simulink model "Active_seat_04_OFFLINE"  (R2017a)
settings: Solver=ode4  StartTime=0.0  StopTime=25  FixedStep=0.005  RelTol=1e-3  EnableMultiTasking=on
undefined symbols (not defined in the file or in its folder): sigbuilder_block
libraries: simulink x8
settings Model: Creator=Stefano  LastModifiedBy=giulio
settings DataIOCC: LimitDataPoints=on
settings OptimizationCC: LifeSpan=inf
settings DebuggingCC: AllowSymbolicDim=off  SFUnexpectedBacktrackingDiag=warning  SFNoUnconditionalDefaultTransitionDiag=warning  SFExecutionAtInitializationDiag=none
settings ModelReferenceCC: PropagateSignalLabelsOutOfModel=off
settings GRTTargetCC: TargetLangStandard=C89/C90 (ANSI)
settings ConfigComp: CovMetricSettings=dw  CovHtmlReporting=on  CovSaveCumulativeToWorkspaceVar=on  CovSaveSingleToWorkspaceVar=on  CovExternalEMLEnable=off

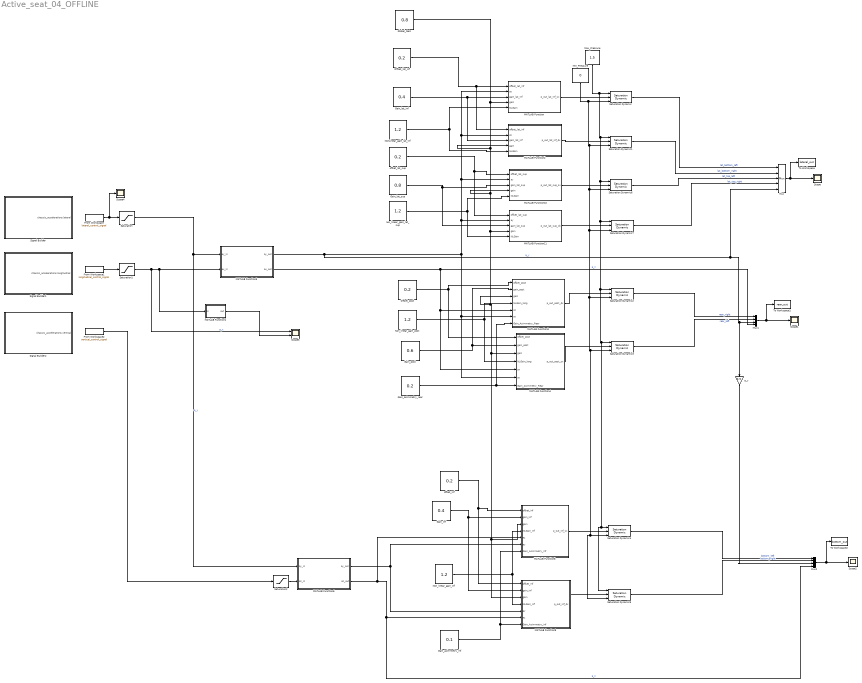
== system Active_seat_04_OFFLINE ==
  From Workspace : FromWorkspace  VariableName=lateral_control_signal  SampleTime=0
  From Workspace1 : FromWorkspace  VariableName=longitudinal_control_signal  SampleTime=0
  From Workspace2 : FromWorkspace  VariableName=vertical_control_signal  SampleTime=0
  Gain_asimmetry_inf : Constant  Value=0.1
  Gain_asimmetry_rear : Constant  Value=0.2
  Gain_inf : Constant  Value=0.4
  Gain_lat_inf : Constant  Value=0.4
  Gain_lat_sup : Constant  Value=0.8
  Gain_post : Constant  Value=0.6
  Global_Gain : Constant  Value=0.8
  MATLAB Function : MATLAB Function  TreatAsAtomicUnit=on
  MATLAB Function1 : MATLAB Function  TreatAsAtomicUnit=on
  MATLAB Function10 : MATLAB Function  TreatAsAtomicUnit=on
  MATLAB Function11 : MATLAB Function  TreatAsAtomicUnit=on
  MATLAB Function2 : MATLAB Function  TreatAsAtomicUnit=on
  MATLAB Function3 : MATLAB Function  TreatAsAtomicUnit=on
  MATLAB Function4 : MATLAB Function  TreatAsAtomicUnit=on
  MATLAB Function5 : MATLAB Function  TreatAsAtomicUnit=on
  MATLAB Function6 : MATLAB Function  TreatAsAtomicUnit=on
  MATLAB Function8 : MATLAB Function  TreatAsAtomicUnit=on
  MATLAB Function9 : MATLAB Function  TreatAsAtomicUnit=on
  Max_Pressure : Constant  Value=1.5
  Min_Pressure : Constant  Value=0
  Mux : Mux  Inputs=5
  Mux1 : Mux
  Mux2 : Mux
  NonLinear_gain_lat_inf : Constant  Value=1.2
  Non_linear_gain_inf : Constant  Value=1.2
  Non_linear_gain_post : Constant  Value=1.2
  Offset_lat_inf : Constant  Value=0.2
  Offset_post : Constant  Value=0.2
  Saturation : Saturate  UpperLimit=5  LowerLimit=-5
  Saturation Dynamic{,1..7} (8 alike) : simulink/Discontinuities/Saturation Dynamic  OutMin=[]  OutMax=[]  OutDataTypeStr=Inherit: Same as second input  OutDataType=fixdt(1, 16)  OutScaling=2^-10  DoSatur=off
  Saturation1 : Saturate  UpperLimit=5  LowerLimit=-5
  Saturation2 : Saturate  UpperLimit=5  LowerLimit=-5
  Scope{,1..2,4} (4 alike) : Scope
  Scope3 : Scope  NumInputPorts=2
  Signal Builder : Subsystem  Tag=STV Subsys  LoadFcn=sigbuilder_block('load');  StartFcn=sigbuilder_block('start');  StopFcn=sigbuilder_block('stop');  ClipboardFcn=sigbuilder_block('clipboard');  mask(Sigbuilder block){tuvar=[0:10]}
      mask help: Simulink:masks:SigbuilderBlock_MD
      mask init:
      | if ~strcmp(get_param(bdroot(gcbh),'SimulationStatus'),'stopped') tuvar = sigbuilder_block('maskInit'); end
      settings: CopyFcn=sigbuilder_block('copy');  DeleteFcn=sigbuilder_block('delete');  ModelCloseFcn=sigbuilder_block('modelClose');  PreSaveFcn=sigbuilder_block('preSave');  PauseFcn=sigbuilder_block('pause');  ContinueFcn=sigbuilder_block('continue');  NameChangeFcn=sigbuilder_block('namechange');  OpenFcn=sigbuilder_block('open',[333 123 550.8 400.2 ]);  CloseFcn=sigbuilder_block('close');
      mask Display: plot(0, 0, 100, 100,[2, 2, 32, 32, 2], [68, 8, 8, 68, 68],[32, 2], [38, 38], [32, 19, 2],[53, 60, 44], [32, 17, 17, 2],[16, 16, 31, 31]);txt = getActiveGroup(gcbh);text(2, 100, txt,'verticalAlignment', 'top');
  Signal Builder1 : Subsystem  Tag=STV Subsys  LoadFcn=sigbuilder_block('load');  StartFcn=sigbuilder_block('start');  StopFcn=sigbuilder_block('stop');  ClipboardFcn=sigbuilder_block('clipboard');  mask(Sigbuilder block){tuvar=[0:10]}
      mask help: Simulink:masks:SigbuilderBlock_MD
      mask init:
      | if ~strcmp(get_param(bdroot(gcbh),'SimulationStatus'),'stopped') tuvar = sigbuilder_block('maskInit'); end
      settings: CopyFcn=sigbuilder_block('copy');  DeleteFcn=sigbuilder_block('delete');  ModelCloseFcn=sigbuilder_block('modelClose');  PreSaveFcn=sigbuilder_block('preSave');  PauseFcn=sigbuilder_block('pause');  ContinueFcn=sigbuilder_block('continue');  NameChangeFcn=sigbuilder_block('namechange');  OpenFcn=sigbuilder_block('open',[333 123 550.8 400.2 ]);  CloseFcn=sigbuilder_block('close');
      mask Display: plot(0, 0, 100, 100,[2, 2, 32, 32, 2], [68, 8, 8, 68, 68],[32, 2], [38, 38], [32, 19, 2],[53, 60, 44], [32, 17, 17, 2],[16, 16, 31, 31]);txt = getActiveGroup(gcbh);text(2, 100, txt,'verticalAlignment', 'top');
  Signal Builder2 : Subsystem  Tag=STV Subsys  LoadFcn=sigbuilder_block('load');  StartFcn=sigbuilder_block('start');  StopFcn=sigbuilder_block('stop');  ClipboardFcn=sigbuilder_block('clipboard');  mask(Sigbuilder block){tuvar=[0:10]}
      mask help: Simulink:masks:SigbuilderBlock_MD
      mask init:
      | if ~strcmp(get_param(bdroot(gcbh),'SimulationStatus'),'stopped') tuvar = sigbuilder_block('maskInit'); end
      settings: CopyFcn=sigbuilder_block('copy');  DeleteFcn=sigbuilder_block('delete');  ModelCloseFcn=sigbuilder_block('modelClose');  PreSaveFcn=sigbuilder_block('preSave');  PauseFcn=sigbuilder_block('pause');  ContinueFcn=sigbuilder_block('continue');  NameChangeFcn=sigbuilder_block('namechange');  OpenFcn=sigbuilder_block('open',[333 123 550.8 400.2 ]);  CloseFcn=sigbuilder_block('close');
      mask Display: plot(0, 0, 100, 100,[2, 2, 32, 32, 2], [68, 8, 8, 68, 68],[32, 2], [38, 38], [32, 19, 2],[53, 60, 44], [32, 17, 17, 2],[16, 16, 31, 31]);txt = getActiveGroup(gcbh);text(2, 100, txt,'verticalAlignment', 'top');
  To Workspace : ToWorkspace  VariableName=lateral_out  SaveFormat=Structure With Time  SampleTime=-1
  To Workspace1 : ToWorkspace  VariableName=rear_out  SaveFormat=Structure With Time  SampleTime=-1
  To Workspace2 : ToWorkspace  VariableName=bottom_out  SaveFormat=Structure With Time  SampleTime=-1
  a_y : Gain  Gain=0.5
  non_linear_gain_lat_sup : Constant  Value=1.2
  offset_inf : Constant  Value=0.2
  offset_lat_sup : Constant  Value=0.2
  wires:
  MATLAB Function2/1(p_out_lat_inf_dx) -> Saturation Dynamic1/2
  MATLAB Function/1(p_out_lat_inf_sx) -> Saturation Dynamic/2
  MATLAB Function3/1(p_out_post_dx) -> Saturation Dynamic2/2
  MATLAB Function4/1(p_out_post_sx) -> Saturation Dynamic3/2
  Gain_lat_inf/1 -> MATLAB Function2/3(gain_lat_inf), MATLAB Function/3(gain_lat_inf)
  MATLAB Function5/2(ax_out) -> Mux1/4, MATLAB Function4/5(ax), MATLAB Function3/5(ax)  "a_x"
  Gain_post/1 -> MATLAB Function4/2(gain_post), MATLAB Function3/2(gain_post)
  Offset_lat_inf/1 -> MATLAB Function2/1(offset_lat_inf), MATLAB Function/1(offset_lat_inf)
  Offset_post/1 -> MATLAB Function4/1(offset_post), MATLAB Function3/1(offset_post)
  Max_Pressure/1 -> Saturation Dynamic/1, Saturation Dynamic6/1, Saturation Dynamic5/1, Saturation Dynamic4/1, Saturation Dynamic3/1, Saturation Dynamic2/1, Saturation Dynamic7/1, Saturation Dynamic1/1
  Min_Pressure/1 -> Saturation Dynamic5/3, Saturation Dynamic4/3, Saturation Dynamic3/3, Saturation Dynamic2/3, Saturation Dynamic7/3, Saturation Dynamic6/3, Saturation Dynamic1/3, Saturation Dynamic/3
  Global_Gain/1 -> MATLAB Function/4(gain), MATLAB Function2/4(gain), MATLAB Function10/4(gain), MATLAB Function11/4(gain), MATLAB Function4/3(gain), MATLAB Function9/3(gain), MATLAB Function8/3(gain), MATLAB Function3/3(gain)
  NonLinear_gain_lat_inf/1 -> MATLAB Function2/5(NLGain), MATLAB Function/5(NLGain)
  Non_linear_gain_post/1 -> MATLAB Function4/4(NLGain_long), MATLAB Function3/4(NLGain_long)
  MATLAB Function6/1(ay_out) -> MATLAB Function9/5(ay), MATLAB Function8/6(ay)
  MATLAB Function6/2(az_out) -> MATLAB Function9/6(az), Mux2/4, MATLAB Function8/5(az)  "a_z"
  offset_inf/1 -> MATLAB Function9/1(offset_inf), MATLAB Function8/1(offset_inf)
  Gain_inf/1 -> MATLAB Function9/2(gain_inf), MATLAB Function8/2(gain_inf)
  Non_linear_gain_inf/1 -> MATLAB Function9/4(NLGain_inf), MATLAB Function8/4(NLGain_inf)
  MATLAB Function8/1(p_out_inf_sx) -> Saturation Dynamic4/2
  MATLAB Function9/1(p_out_inf_dx) -> Saturation Dynamic5/2
  Saturation Dynamic/1 -> Mux/1  "lat_bottom_left"
  Gain_asimmetry_rear/1 -> MATLAB Function4/7(Gain_Asimmetry_Rear), MATLAB Function3/7(Gain_Asimmetry_Rear)
  Gain_asimmetry_inf/1 -> MATLAB Function9/7(Gain_Asimmetry_Inf), MATLAB Function8/7(Gain_Asimmetry_Inf)
  offset_lat_sup/1 -> MATLAB Function11/1(offset_lat_sup), MATLAB Function10/1(offset_lat_sup)
  Gain_lat_sup/1 -> MATLAB Function11/3(gain_lat_sup), MATLAB Function10/3(gain_lat_sup)
  non_linear_gain_lat_sup/1 -> MATLAB Function11/5(NLGain), MATLAB Function10/5(NLGain)
  MATLAB Function10/1(p_out_lat_sup_sx) -> Saturation Dynamic6/2
  MATLAB Function11/1(p_out_lat_sup_dx) -> Saturation Dynamic7/2
  Saturation Dynamic6/1 -> Mux/3  "lat_top_left"
  Saturation Dynamic3/1 -> Mux1/2  "rear_left"
  Saturation Dynamic2/1 -> Mux1/1  "rear_right"
  Saturation Dynamic7/1 -> Mux/4  "lat_top_right"
  Saturation Dynamic1/1 -> Mux/2  "lat_bottom_right"
  Saturation2/1 -> MATLAB Function6/2(az_in)
  MATLAB Function5/1(ay_out) -> Mux/5, a_y/1, Mux1/3, MATLAB Function11/2(ay), MATLAB Function10/2(ay), MATLAB Function2/2(ay), MATLAB Function/2(ay), MATLAB Function4/6(ay), MATLAB Function3/6(ay)  "a_y"
  Saturation Dynamic5/1 -> Mux2/2  "bottom_right"
  Saturation Dynamic4/1 -> Mux2/1  "bottom_left"
  Mux/1 -> To Workspace/1, Scope/1
  Mux1/1 -> To Workspace1/1, Scope1/1
  Mux2/1 -> To Workspace2/1, Scope2/1
  Saturation1/1 -> Scope3/1, MATLAB Function1/1(in), MATLAB Function5/2(ax_in)  "a_x"
  Saturation/1 -> MATLAB Function5/1(ay_in), MATLAB Function6/1(ay_in)  "a_y"
  a_y/1 -> Mux2/3
  MATLAB Function1/1(out) -> Scope3/2
  From Workspace/1 -> Scope4/1, Saturation/1
  From Workspace1/1 -> Saturation1/1
  From Workspace2/1 -> Saturation2/1

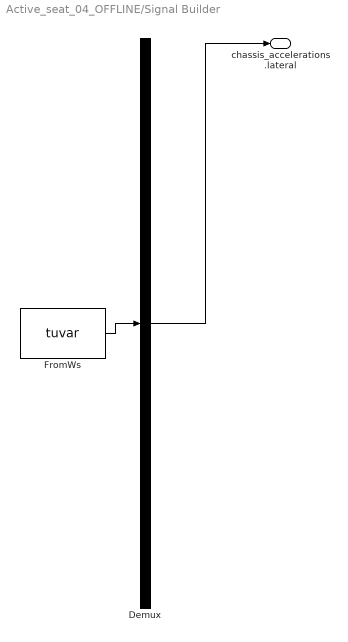
== system Active_seat_04_OFFLINE/Signal Builder ==
  Demux : Demux  Tag=STV Demux  Outputs=1
  FromWs : FromWorkspace  Tag=STV FromWs  VariableName=tuvar  SampleTime=0
      SigBuilderData=|
      | common.afterFinalStr = 'Extrapolate'
      | common.sampleTime = 0
      | dataSet.timeRange = [0 20]
      | dataSet.name = 'Sheet2'
      | sbobj.Name = 'Signal Builder'
      | sbobj.Groups.Name = 'Sheet2'
      | sbobj.Groups.Signals.Name = 'chassis_accelerations.lateral'
      | sbobj.Groups.Signals.XData = [0 0.01 0.02 0.03 0.04 0.05 0.06 0.07 0.08 0.09 0.1 0.11 ... (2001 elements, 1x2001)]
      | sbobj.Groups.Signals.YData = [0.000478634655 0.000129276232 3.6072942e-05 -2.112549e-05 -7.1603792e-05 -0.000121279107 -0.000175679346 -0.000234885552 -0.000306858954 -0.000391455114 -0.000499574859 -0.000629629793 ... (2001 elements, 1x2001)]
      | sbobj.Groups.TimeRange = [0 20]
  chassis_accelerations.lateral : Outport
  wires:
  Demux/1 -> chassis_accelerations.lateral/1
  FromWs/1 -> Demux/1

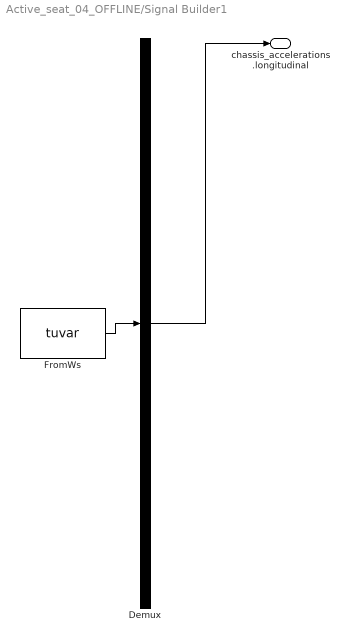
== system Active_seat_04_OFFLINE/Signal Builder1 ==
  Demux : Demux  Tag=STV Demux  Outputs=1
  FromWs : FromWorkspace  Tag=STV FromWs  VariableName=tuvar  SampleTime=0
      SigBuilderData=|
      | common.afterFinalStr = 'Extrapolate'
      | common.sampleTime = 0
      | dataSet.timeRange = [0 20]
      | dataSet.name = 'Longitudinal'
      | sbobj.Name = 'Signal Builder'
      | sbobj.Groups.Name = 'Longitudinal'
      | sbobj.Groups.Signals.Name = 'chassis_accelerations.longitudinal'
      | sbobj.Groups.Signals.XData = [0 0.01 0.02 0.03 0.04 0.05 0.06 0.07 0.08 0.09 0.1 0.11 ... (2001 elements, 1x2001)]
      | sbobj.Groups.Signals.YData = [0.058278837648 -0.089374338918 -0.030931761392 -0.011216646147 -0.00509287137 -0.003559304464 -0.003430377764 -0.003599319044 -0.003706593044 -0.00366417199 -0.003481530457 -0.00319927602 ... (2001 elements, 1x2001)]
      | sbobj.Groups.TimeRange = [0 20]
  chassis_accelerations.longitudinal : Outport
  wires:
  Demux/1 -> chassis_accelerations.longitudinal/1
  FromWs/1 -> Demux/1

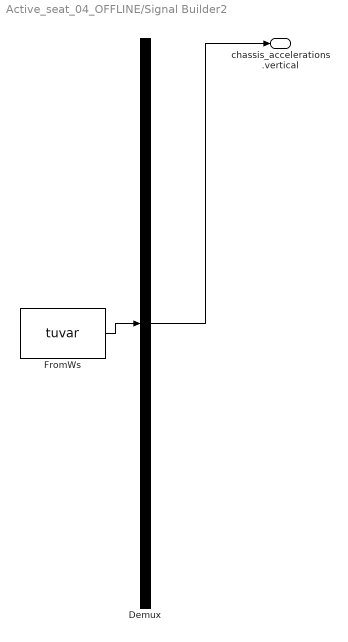
== system Active_seat_04_OFFLINE/Signal Builder2 ==
  Demux : Demux  Tag=STV Demux  Outputs=1
  FromWs : FromWorkspace  Tag=STV FromWs  VariableName=tuvar  SampleTime=0
      SigBuilderData=|
      | common.afterFinalStr = 'Extrapolate'
      | common.sampleTime = 0
      | dataSet.timeRange = [0 13.23]
      | dataSet.name = 'Sheet2'
      | sbobj.Name = 'Signal Builder'
      | sbobj.Groups.Name = 'Sheet2'
      | sbobj.Groups.Signals.Name = 'chassis_accelerations.vertical'
      | sbobj.Groups.Signals.XData = [0 0.01 0.02 0.03 0.04 0.05 0.06 0.07 0.08 0.09 0.1 0.11 ... (1324 elements, 1x1324)]
      | sbobj.Groups.Signals.YData = [0.04903169739 0.02864196724 -0.005041723995 -0.034616068594 -0.049603443105 -0.035547620678 -0.010103069315 0.020982459823 0.069002335908 0.130313504211 0.194446293912 0.261755400015 ... (1324 elements, 1x1324)]
      | sbobj.Groups.TimeRange = [0 13.23]
  chassis_accelerations.vertical : Outport
  wires:
  Demux/1 -> chassis_accelerations.vertical/1
  FromWs/1 -> Demux/1

== matlab function Active_seat_04_OFFLINE/MATLAB Function1 ==
  data: in input; out output
function out = fcn(in)
%#codegen

fc = 300;
fs = 1000;

[b,a] = butter(6,fc/(fs/2));
%freqz(b,a);

out = filter (b,a, in);

== matlab function Active_seat_04_OFFLINE/MATLAB Function ==
  data: offset_lat_inf input; ay input; p_out_lat_inf_sx output; gain_lat_inf input; gain input; NLGain input
function p_out_lat_inf_sx = lat_inf_sx(offset_lat_inf, ay, gain_lat_inf, gain, NLGain)
%#codegen


p_out_lat_inf_sx = offset_lat_inf + gain*sign(ay)*abs(ay)^NLGain*gain_lat_inf;

== matlab function Active_seat_04_OFFLINE/MATLAB Function2 ==
  data: offset_lat_inf input; ay input; p_out_lat_inf_dx output; gain_lat_inf input; gain input; NLGain input
function p_out_lat_inf_dx = lat_inf_dx(offset_lat_inf, ay, gain_lat_inf, gain, NLGain)
%#codegen


p_out_lat_inf_dx = offset_lat_inf - gain*sign(ay)*abs(ay)^NLGain*gain_lat_inf;

== matlab function Active_seat_04_OFFLINE/MATLAB Function3 ==
  data: offset_post input; p_out_post_dx output; gain_post input; gain input; NLGain_long input; ax input; ay input; Gain_Asimmetry_Rear input
function p_out_post_dx = post_dx(offset_post, gain_post, gain, NLGain_long, ax, ay, Gain_Asimmetry_Rear)
%#codegen


b = offset_post + sign(ax)*abs(ax)^NLGain_long*gain*gain_post;

p_out_post_dx = b-b*Gain_Asimmetry_Rear*2/pi*atan(ay/abs(ax));

== matlab function Active_seat_04_OFFLINE/MATLAB Function4 ==
  data: offset_post input; p_out_post_sx output; gain_post input; gain input; NLGain_long input; ax input; ay input; Gain_Asimmetry_Rear input
function p_out_post_sx = post_sx(offset_post, gain_post, gain, NLGain_long, ax, ay, Gain_Asimmetry_Rear)
%#codegen


b = offset_post + sign(ax)*abs(ax)^NLGain_long*gain*gain_post;

p_out_post_sx = b+b*Gain_Asimmetry_Rear*2/pi*atan(ay/abs(ax));

== matlab function Active_seat_04_OFFLINE/MATLAB Function5 ==
  data: ay_out output; ay_in input; ax_in input; ax_out output; filter_pars parameter
%#codegen
function [ay_out, ax_out] = acceleration_filter(ay_in, ax_in, filter_pars)
% [ax_out, ay_out] = acceleration_filter(ax_in, ay_in, pars)
% Inputs:
% - ax_in : longitudinal acceleration
% - ay_in : lateral acceleration
% - filter_pars.fcx : longitudinal cutt-off frequency
% - filter_pars.fcy : lateral cutt-off frequency
% - filter_pars.Ts  : sampling time
% Outputs:
% - ax_out : filtered longitudinal acceleration
% - ay_out : filtered lateral acceleration

persistent ax_state ay_state; % filter state variables
persistent Ax Bx Cx Dx; % longitudinal filter coefficients
persistent Ay By Cy Dy; % lateral filter coefficients

if isempty(ax_state)
    ax_state = 0;
    ay_state = 0;
    [Ax,Bx,Cx,Dx] = butter1_lp(2*pi*filter_pars.fcx, filter_pars.Ts);
    [Ay,By,Cy,Dy] = butter1_lp(2*pi*filter_pars.fcy, filter_pars.Ts);
end

ax_state = Ax*ax_state + Bx*ax_in;
ax_out = Cx*ax_state + Dx*ax_in;
ay_state = Ay*ay_state + By*ay_in;
ay_out = Cy*ay_state + Dy*ay_in;

function [A,B,C,D] = butter1_lp(wc,Ts)
% Butterworth filter of first order (identical to MatLab [fA,fB,fC,fD] = butter(1,wc/2/pi*Ts*2))

if wc==0 
    A = [0]; 
    B = [0];
    C = [0];
    D = 0;
else
    B0=1;
    B2 = 0;
    B1=1;
    A0 = 1;
    A1 = 0;
    A2 = 0;
    C = 1 / tan( wc/2*Ts );
    A = B0 + B1*C + B2*C^2;
    a0 = ( A0 + A1*C  )/A;
    a1 = ( A0 + A1*C ) / A;
    b1 = ( B0 - B1* C  ) / A;

    a0c = a0;
    a1c = a1-b1*a0;

    A = [-b1]; 
    B = [1];
    C = [a1c];
    D = a0c;
end

== matlab function Active_seat_04_OFFLINE/MATLAB Function6 ==
  data: ay_out output; ay_in input; az_in input; az_out output; filter_pars parameter
%#codegen
function [ay_out, az_out] = acceleration_filter(ay_in, az_in, filter_pars)
% [ax_out, ay_out] = acceleration_filter(ax_in, ay_in, pars)
% Inputs:
% - ax_in : vertical acceleration
% - ay_in : lateral acceleration
% - filter_pars.fcz : vertical cutt-off frequency
% - filter_pars.fcy : lateral cutt-off frequency
% - filter_pars.Ts  : sampling time
% Outputs:
% - az_out : filtered vertical acceleration
% - ay_out : filtered lateral acceleration

persistent az_state ay_state; % filter state variables
persistent Az Bz Cz Dz; % vertical filter coefficients
persistent Ay By Cy Dy; % lateral filter coefficients

if isempty(az_state)
    az_state = 0;
    ay_state = 0;
    [Az,Bz,Cz,Dz] = butter1_lp(2*pi*filter_pars.fcz, filter_pars.Ts);
    [Ay,By,Cy,Dy] = butter1_lp(2*pi*filter_pars.fcy, filter_pars.Ts);
end

az_state = Az*az_state + Bz*az_in;
az_out = Cz*az_state + Dz*az_in;
ay_state = Ay*ay_state + By*ay_in;
ay_out = Cy*ay_state + Dy*ay_in;

function [A,B,C,D] = butter1_lp(wc,Ts)
% Butterworth filter of first order (identical to MatLab [fA,fB,fC,fD] = butter(1,wc/2/pi*Ts*2))

if wc==0 
    A = [0]; 
    B = [0];
    C = [0];
    D = 0;
else
    B0=1;
    B2 = 0;
    B1=1;
    A0 = 1;
    A1 = 0;
    A2 = 0;
    C = 1 / tan( wc/2*Ts );
    A = B0 + B1*C + B2*C^2;
    a0 = ( A0 + A1*C  )/A;
    a1 = ( A0 + A1*C ) / A;
    b1 = ( B0 - B1* C  ) / A;

    a0c = a0;
    a1c = a1-b1*a0;

    A = [-b1]; 
    B = [1];
    C = [a1c];
    D = a0c;
end

== matlab function Active_seat_04_OFFLINE/MATLAB Function8 ==
  data: offset_inf input; p_out_inf_sx output; gain_inf input; gain input; NLGain_inf input; az input; ay input; Gain_Asimmetry_Inf input
function p_out_inf_sx = inf_sx(offset_inf, gain_inf, gain, NLGain_inf, az, ay, Gain_Asimmetry_Inf)
%#codegen


b = offset_inf + sign(az)*abs(az)^NLGain_inf*gain*gain_inf;

p_out_inf_sx = b + b*Gain_Asimmetry_Inf*2/pi*atan(ay/abs(az));

== matlab function Active_seat_04_OFFLINE/MATLAB Function9 ==
  data: offset_inf input; p_out_inf_dx output; gain_inf input; gain input; NLGain_inf input; ay input; az input; Gain_Asimmetry_Inf input
function p_out_inf_dx = inf_dx(offset_inf, gain_inf, gain, NLGain_inf, ay, az, Gain_Asimmetry_Inf)
%#codegen


b = offset_inf + sign(az)*abs(az)^NLGain_inf*gain*gain_inf;

p_out_inf_dx = b - b*Gain_Asimmetry_Inf*2/pi*atan(ay/abs(az));

== matlab function Active_seat_04_OFFLINE/MATLAB Function10 ==
  data: offset_lat_sup input; ay input; p_out_lat_sup_sx output; gain_lat_sup input; gain input; NLGain input
function p_out_lat_sup_sx = lat_sup_sx(offset_lat_sup, ay, gain_lat_sup, gain, NLGain)
%#codegen


p_out_lat_sup_sx = offset_lat_sup + gain*sign(ay)*abs(ay)^NLGain*gain_lat_sup;

== matlab function Active_seat_04_OFFLINE/MATLAB Function11 ==
  data: offset_lat_sup input; ay input; p_out_lat_sup_dx output; gain_lat_sup input; gain input; NLGain input
function p_out_lat_sup_dx = lat_sup_dx(offset_lat_sup, ay, gain_lat_sup, gain, NLGain)
%#codegen


p_out_lat_sup_dx = offset_lat_sup - gain*sign(ay)*abs(ay)^NLGain*gain_lat_sup;
